simulink model "math_filter"  (R2023a)
settings: Solver=VariableStepAuto  StartTime=0.0  StopTime=10  RelTol=1e-3
settings Model: Creator=belov  LastModifiedBy=belov

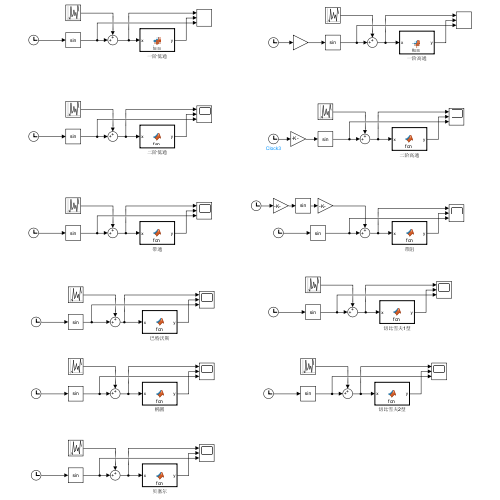
[thumbnail: Simulink's stored preview of the top-level diagram]
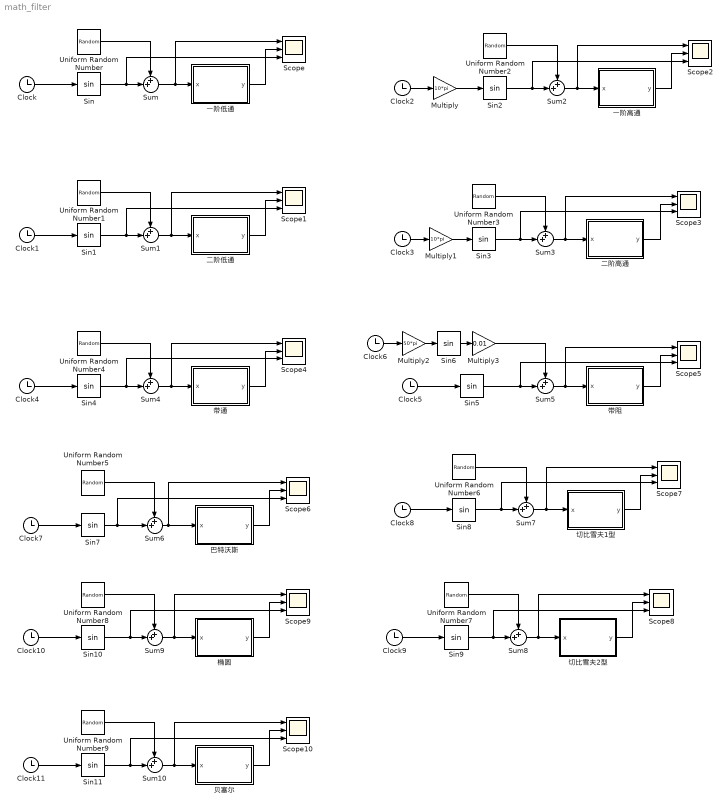
== system math_filter ==
  Clock{,1..11} (12 alike) : Clock
  Multiply : Gain  Gain=10*pi
  Multiply1 : Gain  Gain=10*pi
  Multiply2 : Gain  Gain=50*pi
  Multiply3 : Gain  Gain=0.01
  Scope{,1..10} (11 alike) : Scope  NumInputPorts=3
  Sin{,1..11} (12 alike) : Trigonometry
  Sum{,1..10} (11 alike) : Sum  Inputs=++|
  Uniform Random Number{,1,4..9} (8 alike) : UniformRandomNumber  Minimum=-0.1  Maximum=0.1  SampleTime=0.001
  Uniform Random Number2 : UniformRandomNumber  Minimum=-0.1  Maximum=0.1  SampleTime=2
  Uniform Random Number3 : UniformRandomNumber  Minimum=-0.1  Maximum=0.1  SampleTime=2
  一阶低通 : MATLAB Function  TreatAsAtomicUnit=on  SystemSampleTime=0.001
  一阶高通 : MATLAB Function  TreatAsAtomicUnit=on  SystemSampleTime=0.001
  二阶低通 : MATLAB Function  TreatAsAtomicUnit=on  SystemSampleTime=0.001
  二阶高通 : MATLAB Function  TreatAsAtomicUnit=on  SystemSampleTime=0.001
  切比雪夫1型 : MATLAB Function  TreatAsAtomicUnit=on  SystemSampleTime=0.001
  切比雪夫2型 : MATLAB Function  TreatAsAtomicUnit=on  SystemSampleTime=0.001
  巴特沃斯 : MATLAB Function  TreatAsAtomicUnit=on  SystemSampleTime=0.001
  带通 : MATLAB Function  TreatAsAtomicUnit=on  SystemSampleTime=0.001
  带阻 : MATLAB Function  TreatAsAtomicUnit=on  SystemSampleTime=0.001
  椭圆 : MATLAB Function  TreatAsAtomicUnit=on  SystemSampleTime=0.001
  贝塞尔 : MATLAB Function  TreatAsAtomicUnit=on  SystemSampleTime=0.001
  wires:
  Clock/1 -> Sin/1
  Uniform Random Number/1 -> Sum/1
  Sin/1 -> Scope/3, Sum/2
  Sum/1 -> Scope/1, 一阶低通/1(x)
  一阶低通/1(y) -> Scope/2
  二阶低通/1(y) -> Scope1/2
  Sum1/1 -> Scope1/1, 二阶低通/1(x)
  Sin1/1 -> Scope1/3, Sum1/2
  Uniform Random Number1/1 -> Sum1/1
  Clock1/1 -> Sin1/1
  Clock2/1 -> Multiply/1
  Sin2/1 -> Scope2/3, Sum2/2
  Uniform Random Number2/1 -> Sum2/1
  Sum2/1 -> Scope2/1, 一阶高通/1(x)
  一阶高通/1(y) -> Scope2/2
  Multiply/1 -> Sin2/1
  Clock3/1 -> Multiply1/1
  Sin3/1 -> Scope3/3, Sum3/2
  Uniform Random Number3/1 -> Sum3/1
  Sum3/1 -> Scope3/1, 二阶高通/1(x)
  二阶高通/1(y) -> Scope3/2
  Multiply1/1 -> Sin3/1
  Clock4/1 -> Sin4/1
  Uniform Random Number4/1 -> Sum4/1
  Sin4/1 -> Scope4/3, Sum4/2
  Sum4/1 -> Scope4/1, 带通/1(x)
  带通/1(y) -> Scope4/2
  带阻/1(y) -> Scope5/2
  Sum5/1 -> Scope5/1, 带阻/1(x)
  Clock5/1 -> Sin5/1
  Sin5/1 -> Scope5/3, Sum5/2
  Sin6/1 -> Multiply3/1
  Clock6/1 -> Multiply2/1
  Multiply2/1 -> Sin6/1
  Multiply3/1 -> Sum5/1
  巴特沃斯/1(y) -> Scope6/2
  Sum6/1 -> Scope6/1, 巴特沃斯/1(x)
  Clock7/1 -> Sin7/1
  Sin7/1 -> Scope6/3, Sum6/2
  Uniform Random Number5/1 -> Sum6/1
  切比雪夫1型/1(y) -> Scope7/2
  Sin8/1 -> Scope7/3, Sum7/2
  Sum7/1 -> Scope7/1, 切比雪夫1型/1(x)
  Uniform Random Number6/1 -> Sum7/1
  Clock8/1 -> Sin8/1
  Uniform Random Number7/1 -> Sum8/1
  Clock9/1 -> Sin9/1
  切比雪夫2型/1(y) -> Scope8/2
  Sin9/1 -> Scope8/3, Sum8/2
  Sum8/1 -> Scope8/1, 切比雪夫2型/1(x)
  Uniform Random Number8/1 -> Sum9/1
  Sin10/1 -> Scope9/3, Sum9/2
  椭圆/1(y) -> Scope9/2
  Clock10/1 -> Sin10/1
  Sum9/1 -> Scope9/1, 椭圆/1(x)
  Sum10/1 -> Scope10/1, 贝塞尔/1(x)
  Uniform Random Number9/1 -> Sum10/1
  Sin11/1 -> Scope10/3, Sum10/2
  Clock11/1 -> Sin11/1
  贝塞尔/1(y) -> Scope10/2

== matlab function math_filter/一阶低通 ==
  data: x input; y output
function y = fcn(x)

w_c = 2;

T = 0.001;

persistent x_n_1 y_n_1
if(isempty(x_n_1))
    x_n_1 = 0;
end
if(isempty(y_n_1))
    y_n_1 = 0;
end

y_n = (-(T * w_c - 2) * y_n_1 + T * w_c * x + T * w_c * x_n_1) / (2 + T * w_c);

y_n_1 = y_n;
x_n_1 = x;

y = y_n;

== matlab function math_filter/一阶高通 ==
  data: x input; y output
function y = fcn(x)

w_c = 1;

T = 0.001;

persistent x_n_1 y_n_1
if(isempty(x_n_1))
    x_n_1 = 0;
end
if(isempty(y_n_1))
    y_n_1 = 0;
end

y_n = (2 * x - 2 * x_n_1 - (T - 2) * y_n_1) / (T + 2);

y_n_1 = y_n;
x_n_1 = x;

y = y_n;

== matlab function math_filter/二阶高通 ==
  data: x input; y output
function y = fcn(x)

w_c = 1;

T = 0.001;

persistent x_n_1 x_n_2 y_n_1 y_n_2
if(isempty(x_n_1))
    x_n_1 = 0;
end
if(isempty(y_n_1))
    y_n_1 = 0;
end
if(isempty(x_n_2))
    x_n_2 = 0;
end
if(isempty(y_n_2))
    y_n_2 = 0;
end

y_n = ((w_c * w_c * 4) * x - ...
      (2 * w_c * w_c * 4) * x_n_1 + ...
      (w_c * w_c * 4) * x_n_2 - ...
      (w_c * w_c * T * T - 2 * w_c * T + 4) * y_n_2 - ...
      (2 * w_c * w_c * T * T - 8) * y_n_1) / (4 + 2 * w_c * T + w_c * w_c * T * T);

y_n_2 = y_n_1;
y_n_1 = y_n;
x_n_2 = x_n_1;
x_n_1 = x;


y = y_n;

== matlab function math_filter/带通 ==
  data: x input; y output
function y = fcn(x)

w_c = 1;
B = 2 / w_c;
T = 0.001;

persistent x_n_1 x_n_2 y_n_1 y_n_2
if(isempty(x_n_1))
    x_n_1 = 0;
end
if(isempty(y_n_1))
    y_n_1 = 0;
end
if(isempty(x_n_2))
    x_n_2 = 0;
end
if(isempty(y_n_2))
    y_n_2 = 0;
end

y_n = (2 * T * w_c * B * (x - x_n_2) - ...
      (4 + T * T * w_c * w_c - 2 * T * B) * y_n_2 - ...
      (2 * T * T * w_c * w_c - 8) * y_n_1) / (4 + 2 * T * B + T * T * w_c * w_c);

y_n_2 = y_n_1;
y_n_1 = y_n;
x_n_2 = x_n_1;
x_n_1 = x;


y = y_n;

== matlab function math_filter/带阻 ==
  data: x input; y output
function y = fcn(x)

w_c = 50 * pi;
T = 0.001;

persistent x_n_1 x_n_2 y_n_1 y_n_2
if(isempty(x_n_1))
    x_n_1 = 0;
end
if(isempty(y_n_1))
    y_n_1 = 0;
end
if(isempty(x_n_2))
    x_n_2 = 0;
end
if(isempty(y_n_2))
    y_n_2 = 0;
end

y_n = ((T * T * w_c * w_c + 4) * x + ...
      (2 * T * T * w_c * w_c - 8) * x_n_1 + ...
      (T * T * w_c * w_c + 4) * x_n_2 - ...
      (w_c * w_c * T * T - 2 * w_c * T + 4) * y_n_2 - ...
      (2 * w_c * w_c * T * T - 8) * y_n_1) / (4 + 2 * w_c * T + w_c * w_c * T * T);

y_n_2 = y_n_1;
y_n_1 = y_n;
x_n_2 = x_n_1;
x_n_1 = x;


y = y_n;

== matlab function math_filter/巴特沃斯 ==
  data: x input; y output
function y = fcn(x)

w_c = 1;
B = 2 / w_c;
T = 0.001;

persistent x_n_1 x_n_2 y_n_1 y_n_2
if(isempty(x_n_1))
    x_n_1 = 0;
end
if(isempty(y_n_1))
    y_n_1 = 0;
end
if(isempty(x_n_2))
    x_n_2 = 0;
end
if(isempty(y_n_2))
    y_n_2 = 0;
end

y_n = 0.1553 * x - 0.3102 * x_n_1 + 0.1549 * x_n_2 + 2.001 * y_n_1 - 1.001 * y_n_2;

y_n_2 = y_n_1;
y_n_1 = y_n;
x_n_2 = x_n_1;
x_n_1 = x;


y = y_n;

== matlab function math_filter/切比雪夫1型 ==
  data: x input; y output
function y = fcn(x)

w_c = 1;
B = 2 / w_c;
T = 0.001;

persistent x_n_1 x_n_2 y_n_1 y_n_2
if(isempty(x_n_1))
    x_n_1 = 0;
end
if(isempty(y_n_1))
    y_n_1 = 0;
end
if(isempty(x_n_2))
    x_n_2 = 0;
end
if(isempty(y_n_2))
    y_n_2 = 0;
end

y_n = 0.07054 * x - 0.1409 * x_n_1 + 0.07039 * x_n_2 + 2.001 * y_n_1 - 1.001 * y_n_2;

y_n_2 = y_n_1;
y_n_1 = y_n;
x_n_2 = x_n_1;
x_n_1 = x;


y = y_n;

== matlab function math_filter/切比雪夫2型 ==
  data: x input; y output
function y = fcn(x)

w_c = 1;
B = 2 / w_c;
T = 0.001;

persistent x_n_1 x_n_2 y_n_1 y_n_2
if(isempty(x_n_1))
    x_n_1 = 0;
end
if(isempty(y_n_1))
    y_n_1 = 0;
end
if(isempty(x_n_2))
    x_n_2 = 0;
end
if(isempty(y_n_2))
    y_n_2 = 0;
end

y_n = 0.3704 * x - 0.7406 * x_n_1 + 0.3702 * x_n_2 + 2 * y_n_1 - 1 * y_n_2;

y_n_2 = y_n_1;
y_n_1 = y_n;
x_n_2 = x_n_1;
x_n_1 = x;


y = y_n;

== matlab function math_filter/二阶低通 ==
  data: x input; y output
function y = fcn(x)

w_c = 2;

T = 0.001;

persistent x_n_1 x_n_2 y_n_1 y_n_2
if(isempty(x_n_1))
    x_n_1 = 0;
end
if(isempty(y_n_1))
    y_n_1 = 0;
end
if(isempty(x_n_2))
    x_n_2 = 0;
end
if(isempty(y_n_2))
    y_n_2 = 0;
end

y_n = ((w_c * w_c * T * T) * x + ...
      (2 * w_c * w_c * T * T) * x_n_1 + ...
      (w_c * w_c * T * T) * x_n_2 - ...
      (w_c * w_c * T * T - 2 * w_c * T + 4) * y_n_2 - ...
      (2 * w_c * w_c * T * T - 8) * y_n_1) / (4 + 2 * w_c * T + w_c * w_c * T * T);

y_n_2 = y_n_1;
y_n_1 = y_n;
x_n_2 = x_n_1;
x_n_1 = x;


y = y_n;

== matlab function math_filter/椭圆 ==
  data: x input; y output
function y = fcn(x)

w_c = 1;
B = 2 / w_c;
T = 0.001;

persistent x_n_1 x_n_2 y_n_1 y_n_2
if(isempty(x_n_1))
    x_n_1 = 0;
end
if(isempty(y_n_1))
    y_n_1 = 0;
end
if(isempty(x_n_2))
    x_n_2 = 0;
end
if(isempty(y_n_2))
    y_n_2 = 0;
end

y_n = 0.3077 * x - 0.6158 * x_n_1 + 0.308 * x_n_2 + 2 * y_n_1 - 1 * y_n_2;

y_n_2 = y_n_1;
y_n_1 = y_n;
x_n_2 = x_n_1;
x_n_1 = x;


y = y_n;

== matlab function math_filter/贝塞尔 ==
  data: x input; y output
function y = fcn(x)

w_c = 1;
B = 2 / w_c;
T = 0.001;

persistent x_n_1 x_n_2 y_n_1 y_n_2
if(isempty(x_n_1))
    x_n_1 = 0;
end
if(isempty(y_n_1))
    y_n_1 = 0;
end
if(isempty(x_n_2))
    x_n_2 = 0;
end
if(isempty(y_n_2))
    y_n_2 = 0;
end

y_n = 2.777e-08 * x + 5.554e-08 * x_n_1 + 2.777e-08 * x_n_2 + 1.999 * y_n_1 - 0.9994 * y_n_2;

y_n_2 = y_n_1;
y_n_1 = y_n;
x_n_2 = x_n_1;
x_n_1 = x;


y = y_n;
